simulink model "model"  (R2016a)
settings: Solver=ode4  StartTime=0.0  StopTime=10  FixedStep=0.001  RelTol=1e-3
settings Model: Creator=Priscilla  LastModifiedBy=Priscilla

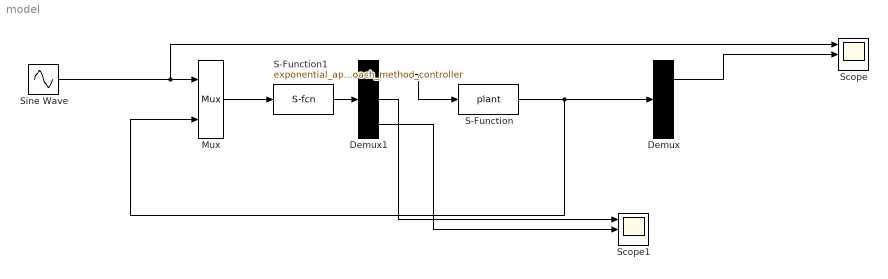
== system model ==
  Demux : Demux  Outputs=2
  Demux1 : Demux  Outputs=3
  Mux : Mux  Inputs=2
  S-Function : S-Function  FunctionName=plant  SFunctionDeploymentMode=off  EnableBusSupport=off
  S-Function1 : S-Function  FunctionName=exponential_approach_method_controller  SFunctionDeploymentMode=off  EnableBusSupport=off
  Scope : Scope  NumInputPorts=3
  Scope1 : Scope  NumInputPorts=3
  Sine Wave : Sin  SampleTime=0
  wires:
  Mux/1 -> S-Function1/1
  Sine Wave/1 -> Scope/1, Mux/1
  S-Function/1 -> Demux/1, Mux/2
  Demux/1 -> Scope/2
  S-Function1/1 -> Demux1/1
  Demux1/1 -> S-Function/1
  Demux1/2 -> Scope1/1
  Demux1/3 -> Scope1/2
